simulink model "sensor_wrapper_harness"  (R2021b)
settings: Solver=VariableStepAuto  StartTime=0.0  StopTime=10.0  RelTol=1e-3
settings Model: DataDictionary=sensor_wrapper.sldd  Creator=ravenst1  LastModifiedBy=timoravensbergen

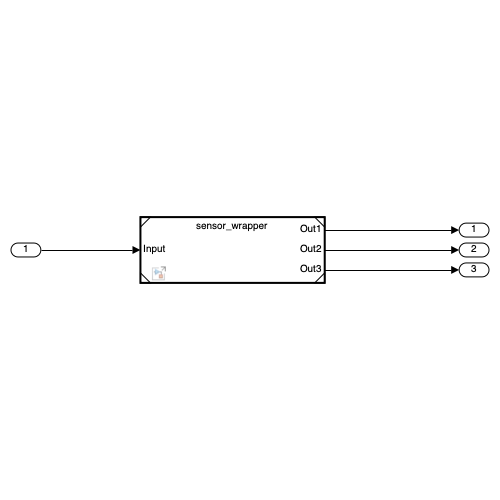
[thumbnail: Simulink's stored preview of the top-level diagram]
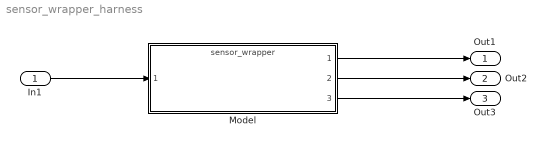
== system sensor_wrapper_harness ==
  In1 : Inport
  Model : ModelReference  ModelNameDialog=sensor_wrapper.slx  SimulationMode=Normal  ModelReferenceVersion=8.3
  Out1 : Outport
  Out2 : Outport  Port=2
  Out3 : Outport  Port=3
  wires:
  In1/1 -> Model/1
  Model/1 -> Out1/1
  Model/2 -> Out2/1
  Model/3 -> Out3/1
